simulink model "CL3DLIPM"  (R2017a)
settings: Solver=VariableStepAuto  StartTime=0.0  StopTime=10.0  RelTol=1e-3
values from neighbouring files (symbols this model uses):
  arm_radius = leg_radius    (= 0.01)    [Nao_paramter.m]
  foot_height = 0.02    [Nao_paramter.m]
  foot_length = 0.1    [Nao_paramter.m]
  foot_mass = 0.17184    [Nao_paramter.m]
  foot_width = 0.05    [Nao_paramter.m]
  ground_height = 0.0025    [Nao_paramter.m]
  ground_length = 5    [Nao_paramter.m]
  ground_width = 2    [Nao_paramter.m]
  hand_mass = 0.18533    [Nao_paramter.m]
  head_mass = 0.60533    [Nao_paramter.m]
  hip_mass = 0.14053    [Nao_paramter.m]
  hip_off_Y = 0.05    [Nao_paramter.m]
  hip_off_Z = 0.085    [Nao_paramter.m]
  leg_radius = 0.01    [Nao_paramter.m]
  lowerarm_length = 0.05595    [Nao_paramter.m]
  lowerarm_mass = 0.07761    [Nao_paramter.m]
  neck_length = 0.03    [Nao_paramter.m]
  neck_mass = 0.07842    [Nao_paramter.m]
  neck_off_Z = 0.1265    [Nao_paramter.m]
  shoulder_mass = 0.09304    [Nao_paramter.m]
  thigh_mass = 0.38968    [Nao_paramter.m]
  tibia_mass = 0.30142    [Nao_paramter.m]
  torso_height = foot_height + tibia_length + thigh_length + 0.5*hip_off_Z    (= 0.2654)    [Nao_paramter.m]
  torso_mass = 1.0496    [Nao_paramter.m]
  upperarm_length = 0.105    [Nao_paramter.m]
  upperarm_mass = 0.15777    [Nao_paramter.m]
undefined symbols (not defined in the file or in its folder): X, Y, Z
libraries: sm_lib x104, nesl_utility x20, Contact_Forces_Lib x10
(part 1 of 4)
settings Model: Creator=zicho  LastModifiedBy=zicho

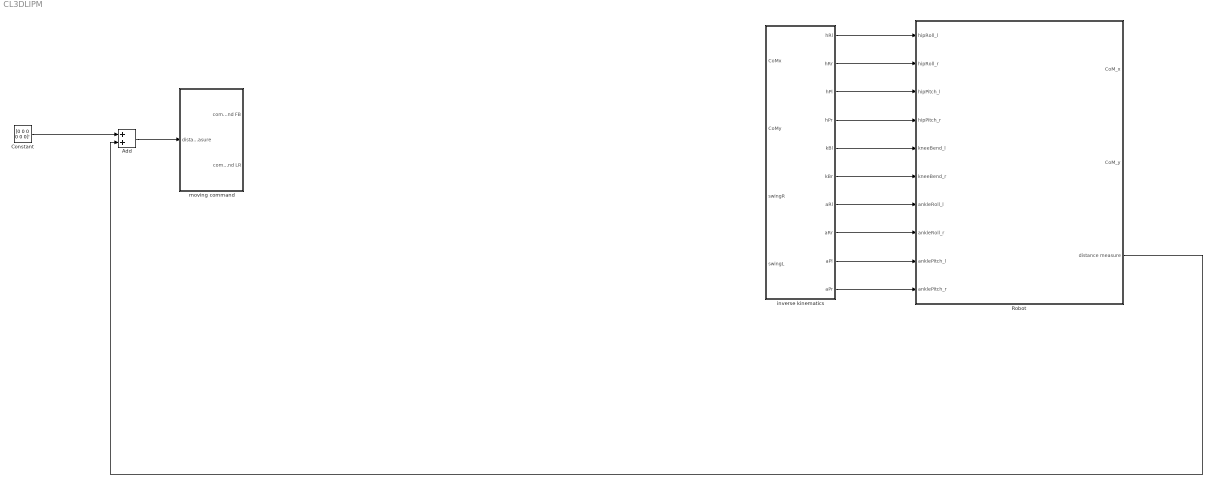
== system CL3DLIPM ==
  Add : Sum
  Constant : Constant  Value=[0 0 0 0 0 0]'  VectorParams1D=off
  "Robot " : Subsystem
      mask Display: image('WeChat Screenshot_20180702161054.png');
  inverse kinematics : Subsystem
  moving command : Subsystem
  wires:
  Constant/1 -> Add/1
  inverse kinematics/1(hRl) -> "Robot "/1(hipRoll_l)
  inverse kinematics/2(hRr) -> "Robot "/2(hipRoll_r)
  inverse kinematics/3(hPl) -> "Robot "/3(hipPitch_l)
  inverse kinematics/4(hPr) -> "Robot "/4(hipPitch_r)
  inverse kinematics/5(kBl) -> "Robot "/5(kneeBend_l)
  inverse kinematics/6(kBr) -> "Robot "/6(kneeBend_r)
  inverse kinematics/7(aRl) -> "Robot "/7(ankleRoll_l)
  inverse kinematics/8(aRr) -> "Robot "/8(ankleRoll_r)
  inverse kinematics/9(aPl) -> "Robot "/9(anklePitch_l)
  inverse kinematics/10(aPr) -> "Robot "/10(anklePitch_r)
  "Robot "/3(distance measure) -> Add/2
  Add/1 -> moving command/1(distance measure)
